simulink model "GeoSurvII_NonLinear_Signal"  (Simulink 7.3)
settings: Solver=ode23  StartTime=0.0  StopTime=30  RelTol=1e-3
values from neighbouring files (symbols this model uses):
  Uo = trim_values(10:13)    [Geo_Find_Trim.m]
  Xo = trim_values(1:9)    [Geo_Find_Trim.m]
undefined symbols (not defined in the file or in its folder): aerosimlib, Earth, sigbuilder_block, WGS
libraries: simulink x3, RCTblocks x1
settings Model: Creator=gblouin  LastModifiedBy=aholtzma
settings OptimizationCC: InitFltsAndDblsToZero=on
settings DebuggingCC: SaveWithParameterizedLinksMsg=none  SignalResolutionControl=TryResolveAllWithWarning  MultiTaskDSMMsg=warning  MultiTaskCondExecSysMsg=none
settings RTWCC: IncludeERTFirstTime=on
settings GRTTargetCC: TargetFcnLib=ansi_tfl_tmw.mat

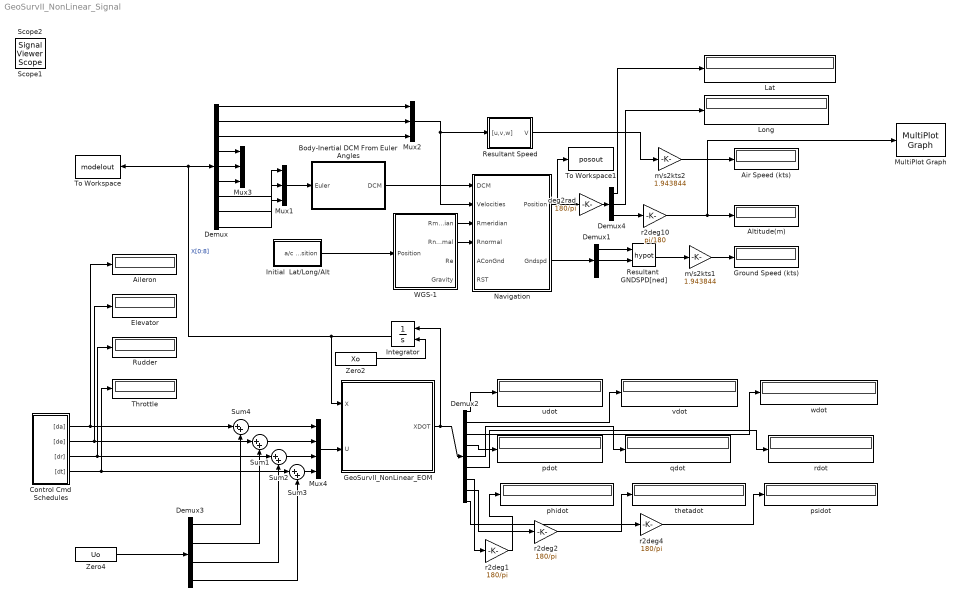
== system GeoSurvII_NonLinear_Signal ==
  Aileron : Display
  Air Speed (kts) : Display
  Altitude(m) : Display
  Body-Inertial DCM From Euler Angles : Subsystem  AncestorBlock=aerosimlib/Transformations/Body-Inertial DCM From Euler Angles
  Control Cmd Schedules : Subsystem
  Demux : Demux  Outputs=9
  Demux1 : Demux  Outputs=3
  Demux2 : Demux  Outputs=9
  Demux3 : Demux
  Demux4 : Demux  Outputs=3
  Elevator : Display
  GeoSurvII_NonLinear_EOM : Stateflow chart
  Ground Speed (kts) : Display
  Initial  Lat/Long/Alt : Subsystem
  Integrator : Integrator  InitialConditionSource=external  InitialCondition=Xo
  Lat : Display
  Long : Display
  MultiPlot Graph : RCTblocks/MultiPlot Graph  Tag=MultiPlot  SystemSampleTime=-1  tmin=0  tmax=60  ymin=450  ymax=550  Tsamp=-1  vnamesave=multisimout
  Mux1 : Mux  Inputs=3
  Mux2 : Mux  Inputs=3
  Mux3 : Mux  Inputs=3
  Mux4 : Mux
  Navigation : Subsystem
  Resultant  GNDSPD[ned] : Math  Operator=hypot  OutDataType=sfix(16)  OutScaling=2^0  SaturateOnIntegerOverflow=on
  Resultant Speed : Subsystem  AncestorBlock=aerosimlib/Equations of Motion/Body-Frame EOM/Kinematics (Euler)
  Rudder : Display
  Sum{1..4} (4 alike) : Sum  Inputs=|++  OutDataType=sfix(16)  OutScaling=2^0
  Throttle : Display
  To Workspace : ToWorkspace  VariableName=modelout  SampleTime=-1  SaveFormat=Structure
  To Workspace1 : ToWorkspace  VariableName=posout  SampleTime=-1  SaveFormat=Structure
  WGS-1 : Subsystem  AncestorBlock=aerosimlib/Earth/WGS-84
  Zero2 : Constant  Value=Xo  OutDataType=sfix(16)  OutScaling=2^0
  Zero4 : Constant  Value=Uo  OutDataType=sfix(16)  OutScaling=2^0
  deg2rad : Gain  Gain=180/pi  ParameterDataType=sfix(16)  ParameterScaling=2^0  OutDataType=sfix(16)  OutScaling=2^0
  m/s2kts1 : Gain  Gain=1.943844  ParameterDataType=sfix(16)  ParameterScaling=2^0  OutDataType=sfix(16)  OutScaling=2^0
  m/s2kts2 : Gain  Gain=1.943844  ParameterDataType=sfix(16)  ParameterScaling=2^0  OutDataType=sfix(16)  OutScaling=2^0
  pdot : Display
  phidot : Display
  psidot : Display
  qdot : Display
  r2deg1 : Gain  Gain=180/pi  ParameterDataType=sfix(16)  ParameterScaling=2^0  OutDataType=sfix(16)  OutScaling=2^0
  r2deg10 : Gain  Gain=pi/180  ParameterDataType=sfix(16)  ParameterScaling=2^0  OutDataType=sfix(16)  OutScaling=2^0
  r2deg2 : Gain  Gain=180/pi  ParameterDataType=sfix(16)  ParameterScaling=2^0  OutDataType=sfix(16)  OutScaling=2^0
  r2deg4 : Gain  Gain=180/pi  ParameterDataType=sfix(16)  ParameterScaling=2^0  OutDataType=sfix(16)  OutScaling=2^0
  rdot : Display
  thetadot : Display
  udot : Display
  vdot : Display
  wdot : Display
  Scope1 : SignalViewerScope  IOType=viewer  NumInputPorts=2  ZoomMode=xonly  RefreshTime=1.500000
      settings: TimeRange=100  YMin=-3.5~-2.84987e-012  YMax=0.5~-2.57845e-012  MaxDataPoints=20000
  Scope2 : SignalViewerScope  IOType=viewer  NumInputPorts=2  ZoomMode=xonly  RefreshTime=1.500000
      settings: TimeRange=100  YMin=-40~9.16954  YMax=10~10.1348  MaxDataPoints=20000
  wires:
  Navigation/1(Position) -> deg2rad/1, To Workspace1/1
  Demux4/1 -> Lat/1
  Demux4/2 -> Long/1
  deg2rad/1 -> Demux4/1
  Demux4/3 -> r2deg10/1
  r2deg10/1 -> Altitude(m)/1, MultiPlot Graph/1
  Navigation/2(Gndspd) -> Demux1/1
  Demux1/1 -> Resultant  GNDSPD[ned]/1
  Demux1/2 -> Resultant  GNDSPD[ned]/2
  Integrator/1 -> GeoSurvII_NonLinear_EOM/1(X), Demux/1, To Workspace/1  "X[0:8]"
  Zero2/1 -> Integrator/2
  Demux2/2 -> vdot/1
  Demux2/1 -> udot/1
  GeoSurvII_NonLinear_EOM/1(XDOT) -> Demux2/1, Integrator/1
  Zero4/1 -> Demux3/1
  Mux4/1 -> GeoSurvII_NonLinear_EOM/2(U)
  Demux/1 -> Mux2/1
  Resultant  GNDSPD[ned]/1 -> m/s2kts1/1
  m/s2kts1/1 -> Ground Speed (kts)/1
  WGS-1/1(Rmeridian) -> Navigation/3(Rmeridian)
  WGS-1/2(Rnormal) -> Navigation/4(Rnormal)
  Body-Inertial DCM From Euler Angles/1(DCM) -> Navigation/1(DCM)
  Mux2/1 -> Navigation/2(Velocities), Resultant Speed/1("[u,v,w]")
  Initial  Lat/Long/Alt/1(a/c Position) -> WGS-1/1(Position)
  Resultant Speed/1(V) -> m/s2kts2/1
  m/s2kts2/1 -> Air Speed (kts)/1
  Demux2/3 -> wdot/1
  Demux2/4 -> pdot/1
  Demux2/5 -> qdot/1
  Demux2/6 -> rdot/1
  Demux2/7 -> r2deg1/1
  r2deg1/1 -> phidot/1
  Demux2/8 -> r2deg2/1
  r2deg2/1 -> thetadot/1
  Demux2/9 -> r2deg4/1
  r2deg4/1 -> psidot/1
  Sum4/1 -> Mux4/1
  Sum1/1 -> Mux4/2
  Sum2/1 -> Mux4/3
  Sum3/1 -> Mux4/4
  Demux3/1 -> Sum4/2
  Demux3/2 -> Sum1/2
  Demux3/3 -> Sum2/2
  Demux3/4 -> Sum3/2
  Demux/2 -> Mux2/2
  Demux/3 -> Mux2/3
  Demux/7 -> Mux1/1
  Demux/8 -> Mux1/2
  Demux/9 -> Mux1/3
  Mux1/1 -> Body-Inertial DCM From Euler Angles/1(Euler)
  Demux/4 -> Mux3/1
  Demux/5 -> Mux3/2
  Demux/6 -> Mux3/3
  Control Cmd Schedules/1("[da]") -> Sum4/1, Aileron/1
  Control Cmd Schedules/2("[de]") -> Sum1/1, Elevator/1
  Control Cmd Schedules/3("[dr]") -> Sum2/1, Rudder/1
  Control Cmd Schedules/4("[dt]") -> Sum3/1, Throttle/1

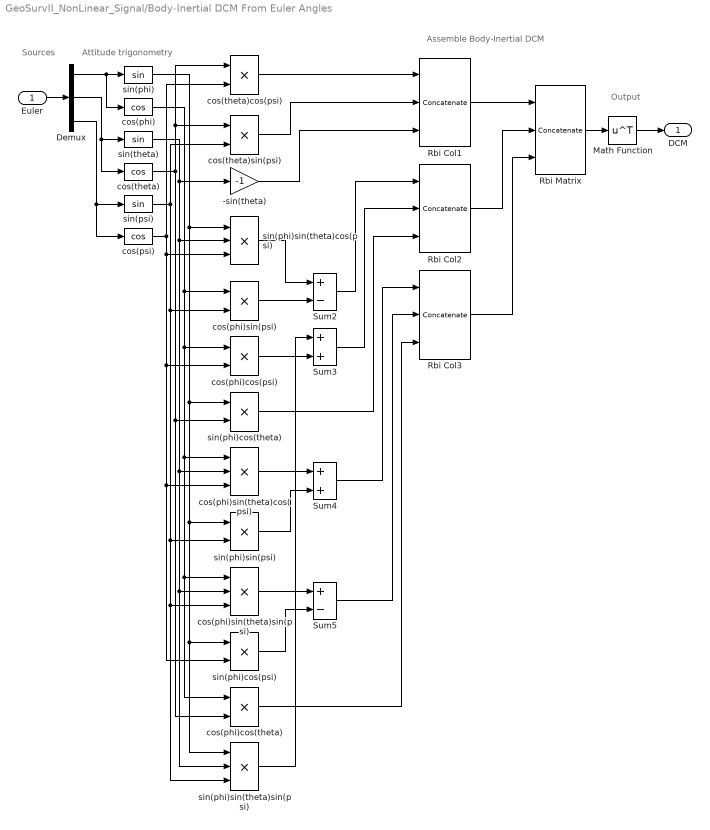
== system GeoSurvII_NonLinear_Signal/Body-Inertial DCM From Euler Angles ==
  note: Sources
  note: Assemble Body-Inertial DCM
  note: Output
  note: Attitude trigonometry
  Euler : Inport  PortDimensions=[3 1]  OutDataType=sfix(16)  OutScaling=2^0
  -sin(theta) : Gain  Gain=-1  ParameterDataType=sfix(16)  ParameterScaling=2^0  OutDataType=sfix(16)  OutScaling=2^0  SaturateOnIntegerOverflow=on  OutDataTypeStr=Inherit: Same as input  ParamDataTypeStr=Inherit: Same as input
  Demux : Demux  Outputs=3
  Math Function : Math  Operator=transpose  OutDataType=sfix(16)  OutScaling=2^0  SaturateOnIntegerOverflow=on
  Rbi Matrix : Concatenate  NumInputs=3  Mode=Multidimensional array  ConcatenateDimension=2
  Rbi Col1 : Concatenate  NumInputs=3  Mode=Multidimensional array
  Rbi Col2 : Concatenate  NumInputs=3  Mode=Multidimensional array
  Rbi Col3 : Concatenate  NumInputs=3  Mode=Multidimensional array
  Sum2 : Sum  Inputs=+-  OutDataType=sfix(16)  OutScaling=2^0  SaturateOnIntegerOverflow=on  InputSameDT=on  OutDataTypeStr=Inherit: Same as first input
  Sum3 : Sum  OutDataType=sfix(16)  OutScaling=2^0  SaturateOnIntegerOverflow=on  InputSameDT=on  OutDataTypeStr=Inherit: Same as first input
  Sum4 : Sum  OutDataType=sfix(16)  OutScaling=2^0  SaturateOnIntegerOverflow=on  InputSameDT=on  OutDataTypeStr=Inherit: Same as first input
  Sum5 : Sum  Inputs=+-  OutDataType=sfix(16)  OutScaling=2^0  SaturateOnIntegerOverflow=on  InputSameDT=on  OutDataTypeStr=Inherit: Same as first input
  cos(phi) : Trigonometry  Operator=cos
  cos(phi)cos(psi) : Product  OutDataType=sfix(16)  OutScaling=2^0  SaturateOnIntegerOverflow=on  InputSameDT=on  OutDataTypeStr=Inherit: Same as first input
  cos(phi)cos(theta) : Product  OutDataType=sfix(16)  OutScaling=2^0  SaturateOnIntegerOverflow=on  InputSameDT=on  OutDataTypeStr=Inherit: Same as first input
  cos(phi)sin(psi) : Product  OutDataType=sfix(16)  OutScaling=2^0  SaturateOnIntegerOverflow=on  InputSameDT=on  OutDataTypeStr=Inherit: Same as first input
  cos(phi)sin(theta)cos(psi) : Product  Inputs=3  OutDataType=sfix(16)  OutScaling=2^0  SaturateOnIntegerOverflow=on  InputSameDT=on  OutDataTypeStr=Inherit: Same as first input
  cos(phi)sin(theta)sin(psi) : Product  Inputs=3  OutDataType=sfix(16)  OutScaling=2^0  SaturateOnIntegerOverflow=on  InputSameDT=on  OutDataTypeStr=Inherit: Same as first input
  cos(psi) : Trigonometry  Operator=cos
  cos(theta) : Trigonometry  Operator=cos
  cos(theta)cos(psi) : Product  OutDataType=sfix(16)  OutScaling=2^0  SaturateOnIntegerOverflow=on  InputSameDT=on  OutDataTypeStr=Inherit: Same as first input
  cos(theta)sin(psi) : Product  OutDataType=sfix(16)  OutScaling=2^0  SaturateOnIntegerOverflow=on  InputSameDT=on  OutDataTypeStr=Inherit: Same as first input
  sin(phi) : Trigonometry
  sin(phi)cos(psi) : Product  OutDataType=sfix(16)  OutScaling=2^0  SaturateOnIntegerOverflow=on  InputSameDT=on  OutDataTypeStr=Inherit: Same as first input
  sin(phi)cos(theta) : Product  OutDataType=sfix(16)  OutScaling=2^0  SaturateOnIntegerOverflow=on  InputSameDT=on  OutDataTypeStr=Inherit: Same as first input
  sin(phi)sin(psi) : Product  OutDataType=sfix(16)  OutScaling=2^0  SaturateOnIntegerOverflow=on  InputSameDT=on  OutDataTypeStr=Inherit: Same as first input
  sin(phi)sin(theta)cos(psi) : Product  Inputs=3  OutDataType=sfix(16)  OutScaling=2^0  SaturateOnIntegerOverflow=on  InputSameDT=on  OutDataTypeStr=Inherit: Same as first input
  sin(phi)sin(theta)sin(psi) : Product  Inputs=3  OutDataType=sfix(16)  OutScaling=2^0  SaturateOnIntegerOverflow=on  InputSameDT=on  OutDataTypeStr=Inherit: Same as first input
  sin(psi) : Trigonometry
  sin(theta) : Trigonometry
  DCM : Outport  OutDataType=sfix(16)  OutScaling=2^0
  wires:
  Euler/1 -> Demux/1
  Rbi Col1/1 -> Rbi Matrix/1
  Rbi Col2/1 -> Rbi Matrix/2
  Rbi Col3/1 -> Rbi Matrix/3
  Rbi Matrix/1 -> Math Function/1
  Demux/1 -> sin(phi)/1, cos(phi)/1
  Demux/2 -> cos(theta)/1, sin(theta)/1
  Demux/3 -> cos(psi)/1, sin(psi)/1
  sin(phi)/1 -> sin(phi)sin(psi)/1, sin(phi)cos(psi)/1, sin(phi)sin(theta)sin(psi)/1, sin(phi)cos(theta)/1, sin(phi)sin(theta)cos(psi)/1
  cos(phi)/1 -> cos(phi)cos(theta)/1, cos(phi)sin(theta)sin(psi)/1, cos(phi)sin(theta)cos(psi)/1, cos(phi)cos(psi)/1, cos(phi)sin(psi)/1
  sin(theta)/1 -> cos(phi)sin(theta)cos(psi)/2, cos(phi)sin(theta)sin(psi)/2, sin(phi)sin(theta)sin(psi)/2, sin(phi)sin(theta)cos(psi)/2, -sin(theta)/1
  cos(theta)/1 -> cos(phi)cos(theta)/2, sin(phi)cos(theta)/2, cos(theta)sin(psi)/1, cos(theta)cos(psi)/1
  sin(psi)/1 -> sin(phi)sin(psi)/2, cos(phi)sin(theta)sin(psi)/3, sin(phi)sin(theta)sin(psi)/3, cos(phi)sin(psi)/2, cos(theta)sin(psi)/2
  cos(psi)/1 -> sin(phi)cos(psi)/2, cos(phi)sin(theta)cos(psi)/3, cos(phi)cos(psi)/2, sin(phi)sin(theta)cos(psi)/3, cos(theta)cos(psi)/2
  cos(phi)sin(psi)/1 -> Sum2/2
  cos(phi)cos(psi)/1 -> Sum3/2
  sin(phi)sin(theta)cos(psi)/1 -> Sum2/1
  cos(phi)sin(theta)cos(psi)/1 -> Sum4/1
  sin(phi)sin(psi)/1 -> Sum4/2
  cos(phi)sin(theta)sin(psi)/1 -> Sum5/1
  sin(phi)cos(psi)/1 -> Sum5/2
  cos(theta)cos(psi)/1 -> Rbi Col1/1
  cos(theta)sin(psi)/1 -> Rbi Col1/2
  -sin(theta)/1 -> Rbi Col1/3
  Sum2/1 -> Rbi Col2/1
  Sum3/1 -> Rbi Col2/2
  sin(phi)cos(theta)/1 -> Rbi Col2/3
  Sum4/1 -> Rbi Col3/1
  Sum5/1 -> Rbi Col3/2
  cos(phi)cos(theta)/1 -> Rbi Col3/3
  Math Function/1 -> DCM/1
  sin(phi)sin(theta)sin(psi)/1 -> Sum3/1

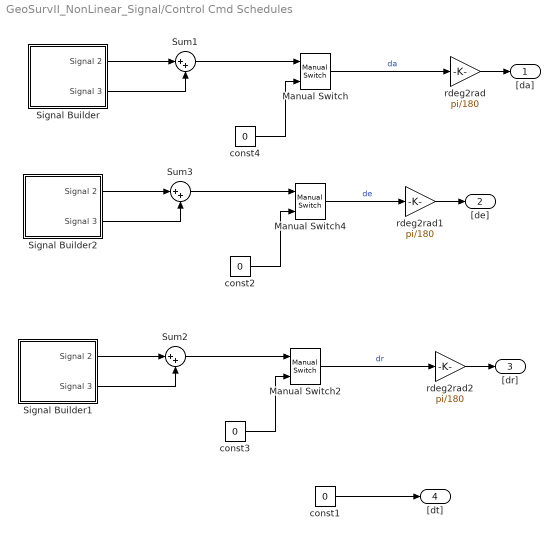
== system GeoSurvII_NonLinear_Signal/Control Cmd Schedules ==
  Manual Switch : simulink/Signal Routing/Manual Switch  SystemSampleTime=-1  sw=0  action=0  varsize=off
  Manual Switch2 : simulink/Signal Routing/Manual Switch  SystemSampleTime=-1  sw=0  action=0  varsize=off
  Manual Switch4 : simulink/Signal Routing/Manual Switch  SystemSampleTime=-1  sw=0  action=0  varsize=off
  Signal Builder : Subsystem  Tag=STV Subsys  LoadFcn=sigbuilder_block('load');  StartFcn=sigbuilder_block('start');  StopFcn=sigbuilder_block('stop');  ClipboardFcn=sigbuilder_block('clipboard');  mask(Sigbuilder block){}
      mask help: Sigbuilder GUI
      mask init:
      | if ~strcmp(get_param(bdroot(gcbh),'SimulationStatus'),'stopped') tuvar = sigbuilder_block('maskInit'); end
      settings: CopyFcn=sigbuilder_block('copy');  DeleteFcn=sigbuilder_block('delete');  ModelCloseFcn=sigbuilder_block('modelClose');  PreSaveFcn=sigbuilder_block('preSave');  NameChangeFcn=sigbuilder_block('namechange');  OpenFcn=sigbuilder_block('open',[6 22.5 948 659.25 ]);  CloseFcn=sigbuilder_block('close');
      mask Display: plot(0,0,100,100,[10,10,40,40,10],[80,20,20,80,80],[40,10],[50,50], [40,27,10],[65,72,56],[40,25,25,10],[28,28,43,43]);
  Signal Builder1 : Subsystem  Tag=STV Subsys  LoadFcn=sigbuilder_block('load');  StartFcn=sigbuilder_block('start');  StopFcn=sigbuilder_block('stop');  ClipboardFcn=sigbuilder_block('clipboard');  mask(Sigbuilder block){}
      mask help: Sigbuilder GUI
      mask init:
      | if ~strcmp(get_param(bdroot(gcbh),'SimulationStatus'),'stopped') tuvar = sigbuilder_block('maskInit'); end
      settings: CopyFcn=sigbuilder_block('copy');  DeleteFcn=sigbuilder_block('delete');  ModelCloseFcn=sigbuilder_block('modelClose');  PreSaveFcn=sigbuilder_block('preSave');  NameChangeFcn=sigbuilder_block('namechange');  OpenFcn=sigbuilder_block('open',[0 19.5 960 695.25 ]);  CloseFcn=sigbuilder_block('close');
      mask Display: plot(0,0,100,100,[10,10,40,40,10],[80,20,20,80,80],[40,10],[50,50], [40,27,10],[65,72,56],[40,25,25,10],[28,28,43,43]);
  Signal Builder2 : Subsystem  Tag=STV Subsys  LoadFcn=sigbuilder_block('load');  StartFcn=sigbuilder_block('start');  StopFcn=sigbuilder_block('stop');  ClipboardFcn=sigbuilder_block('clipboard');  mask(Sigbuilder block){}
      mask help: Sigbuilder GUI
      mask init:
      | if ~strcmp(get_param(bdroot(gcbh),'SimulationStatus'),'stopped') tuvar = sigbuilder_block('maskInit'); end
      settings: CopyFcn=sigbuilder_block('copy');  DeleteFcn=sigbuilder_block('delete');  ModelCloseFcn=sigbuilder_block('modelClose');  PreSaveFcn=sigbuilder_block('preSave');  NameChangeFcn=sigbuilder_block('namechange');  OpenFcn=sigbuilder_block('open',[6 22.5 948 659.25 ]);  CloseFcn=sigbuilder_block('close');
      mask Display: plot(0,0,100,100,[10,10,40,40,10],[80,20,20,80,80],[40,10],[50,50], [40,27,10],[65,72,56],[40,25,25,10],[28,28,43,43]);
  Sum1 : Sum  Inputs=|++  OutDataType=sfix(16)  OutScaling=2^0
  Sum2 : Sum  Inputs=|++  OutDataType=sfix(16)  OutScaling=2^0
  Sum3 : Sum  Inputs=|++  OutDataType=sfix(16)  OutScaling=2^0
  const{1..4} (4 alike) : Constant  Value=0  OutDataType=sfix(16)  OutScaling=2^0
  rdeg2rad : Gain  Gain=pi/180  ParameterDataType=sfix(16)  ParameterScaling=2^0  OutDataType=sfix(16)  OutScaling=2^0
  rdeg2rad1 : Gain  Gain=pi/180  ParameterDataType=sfix(16)  ParameterScaling=2^0  OutDataType=sfix(16)  OutScaling=2^0
  rdeg2rad2 : Gain  Gain=pi/180  ParameterDataType=sfix(16)  ParameterScaling=2^0  OutDataType=sfix(16)  OutScaling=2^0
  "[da]" : Outport  OutDataType=sfix(16)  OutScaling=2^0
  "[de]" : Outport  Port=2  OutDataType=sfix(16)  OutScaling=2^0
  "[dr]" : Outport  Port=3  OutDataType=sfix(16)  OutScaling=2^0
  "[dt]" : Outport  Port=4  OutDataType=sfix(16)  OutScaling=2^0
  wires:
  Signal Builder/1(Signal 2) -> Sum1/1
  Signal Builder/2(Signal 3) -> Sum1/2
  Manual Switch/1 -> rdeg2rad/1  "da"
  Sum1/1 -> Manual Switch/1
  const4/1 -> Manual Switch/2
  Signal Builder1/1(Signal 2) -> Sum2/1
  Signal Builder1/2(Signal 3) -> Sum2/2
  Manual Switch2/1 -> rdeg2rad2/1  "dr"
  Sum2/1 -> Manual Switch2/1
  const3/1 -> Manual Switch2/2
  Signal Builder2/1(Signal 2) -> Sum3/1
  Signal Builder2/2(Signal 3) -> Sum3/2
  Manual Switch4/1 -> rdeg2rad1/1  "de"
  Sum3/1 -> Manual Switch4/1
  const2/1 -> Manual Switch4/2
  const1/1 -> "[dt]"/1
  rdeg2rad/1 -> "[da]"/1
  rdeg2rad1/1 -> "[de]"/1
  rdeg2rad2/1 -> "[dr]"/1

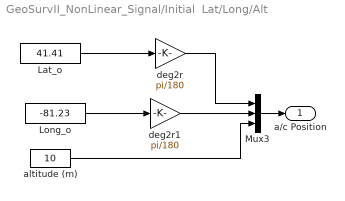
== system GeoSurvII_NonLinear_Signal/Initial  Lat/Long/Alt ==
  Lat_o : Constant  Value=41.41  OutDataType=sfix(16)  OutScaling=2^0
  Long_o : Constant  Value=-81.23  OutDataType=sfix(16)  OutScaling=2^0
  Mux3 : Mux  Inputs=3
  altitude (m) : Constant  Value=10  OutDataType=sfix(16)  OutScaling=2^0
  deg2r : Gain  Gain=pi/180  ParameterDataType=sfix(16)  ParameterScaling=2^0  OutDataType=sfix(16)  OutScaling=2^0
  deg2r1 : Gain  Gain=pi/180  ParameterDataType=sfix(16)  ParameterScaling=2^0  OutDataType=sfix(16)  OutScaling=2^0
  a/c Position : Outport  OutDataType=sfix(16)  OutScaling=2^0
  wires:
  Mux3/1 -> a/c Position/1
  altitude (m)/1 -> Mux3/3
  deg2r1/1 -> Mux3/2
  deg2r/1 -> Mux3/1
  Long_o/1 -> deg2r1/1
  Lat_o/1 -> deg2r/1

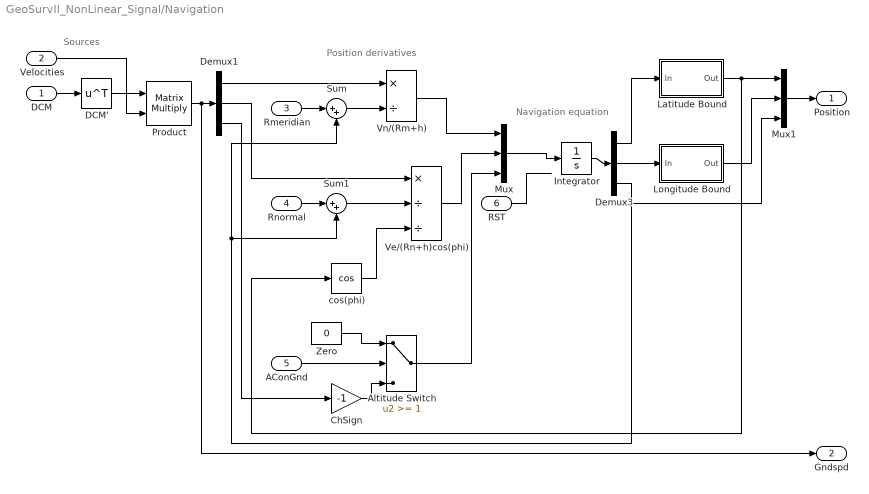
== system GeoSurvII_NonLinear_Signal/Navigation ==
  note: Navigation equation
  note: Position derivatives
  note: Sources
  DCM : Inport  PortDimensions=[3 3]  OutDataType=sfix(16)  OutScaling=2^0
  Velocities : Inport  Port=2  PortDimensions=[3 1]  OutDataType=sfix(16)  OutScaling=2^0
  Rmeridian : Inport  Port=3  PortDimensions=1  OutDataType=sfix(16)  OutScaling=2^0
  Rnormal : Inport  Port=4  PortDimensions=1  OutDataType=sfix(16)  OutScaling=2^0
  AConGnd : Inport  Port=5  PortDimensions=1  OutDataType=sfix(16)  OutScaling=2^0
  RST : Inport  Port=6  PortDimensions=1  OutDataType=sfix(16)  OutScaling=2^0
  Altitude Switch : Switch  Threshold=1  SaturateOnIntegerOverflow=on  InputSameDT=on
  ChSign : Gain  Gain=-1  ParameterDataType=sfix(16)  ParameterScaling=2^0  OutDataType=sfix(16)  OutScaling=2^0  SaturateOnIntegerOverflow=on  OutDataTypeStr=Inherit: Same as input  ParamDataTypeStr=Inherit: Same as input
  DCM' : Math  Operator=transpose  OutDataType=sfix(16)  OutScaling=2^0  SaturateOnIntegerOverflow=on
  Demux1 : Demux  Outputs=3
  Demux3 : Demux  Outputs=3
  Integrator : Integrator  InitialCondition=[41.684028*pi/180 -81.389750*pi/180 500]
  Latitude Bound : Subsystem
      mask Type: Latitude bound
      mask Description: Bounds the latitude to [-pi/2, pi/2]. When the lower bound is exceeded the latitude is increasing again; when the upper bound is exceeded the latitude is decreasing.
  Longitude Bound : Subsystem
      mask Type: Longitude bound
      mask Description: Bounds the longitude to [-pi, pi]. When -pi bound is exceeded the longitude wraps back to pi; when the pi bound is exceeded the longitude wraps back to -pi.
  Mux : Mux  Inputs=3
  Mux1 : Mux  Inputs=3
  Product : Product  Multiplication=Matrix(*)  OutDataType=sfix(16)  OutScaling=2^0  SaturateOnIntegerOverflow=on  InputSameDT=on  OutDataTypeStr=Inherit: Same as first input
  Sum : Sum  Inputs=|++  OutDataType=sfix(16)  OutScaling=2^0  SaturateOnIntegerOverflow=on  InputSameDT=on  OutDataTypeStr=Inherit: Same as first input
  Sum1 : Sum  Inputs=|++  OutDataType=sfix(16)  OutScaling=2^0  SaturateOnIntegerOverflow=on  InputSameDT=on  OutDataTypeStr=Inherit: Same as first input
  Ve/(Rn+h)cos(phi) : Product  Inputs=*//  OutDataType=sfix(16)  OutScaling=2^0  SaturateOnIntegerOverflow=on  InputSameDT=on  OutDataTypeStr=Inherit: Same as first input
  Vn/(Rm+h) : Product  Inputs=*/  OutDataType=sfix(16)  OutScaling=2^0  SaturateOnIntegerOverflow=on  InputSameDT=on  OutDataTypeStr=Inherit: Same as first input
  Zero : Constant  Value=0  OutDataType=sfix(16)  OutScaling=2^0
  cos(phi) : Trigonometry  Operator=cos
  Position : Outport  OutDataType=sfix(16)  OutScaling=2^0
  Gndspd : Outport  Port=2  OutDataType=sfix(16)  OutScaling=2^0
  wires:
  Latitude Bound/1(Out) -> Mux1/1, cos(phi)/1
  Mux1/1 -> Position/1
  Longitude Bound/1(Out) -> Mux1/2
  Demux3/1 -> Latitude Bound/1(In)
  Demux3/2 -> Longitude Bound/1(In)
  Demux3/3 -> Mux1/3, Sum1/2, Sum/2
  cos(phi)/1 -> Ve/(Rn+h)cos(phi)/3
  Integrator/1 -> Demux3/1
  RST/1 -> ?
  Mux/1 -> Integrator/1
  Altitude Switch/1 -> Mux/3
  ChSign/1 -> Altitude Switch/3
  Zero/1 -> Altitude Switch/1
  AConGnd/1 -> Altitude Switch/2
  DCM'/1 -> Product/1
  DCM/1 -> DCM'/1
  Ve/(Rn+h)cos(phi)/1 -> Mux/2
  Sum1/1 -> Ve/(Rn+h)cos(phi)/2
  Vn/(Rm+h)/1 -> Mux/1
  Sum/1 -> Vn/(Rm+h)/2
  Rnormal/1 -> Sum1/1
  Rmeridian/1 -> Sum/1
  Product/1 -> Gndspd/1, Demux1/1
  Demux1/2 -> Ve/(Rn+h)cos(phi)/1
  Demux1/3 -> ChSign/1
  Demux1/1 -> Vn/(Rm+h)/1
  Velocities/1 -> Product/2

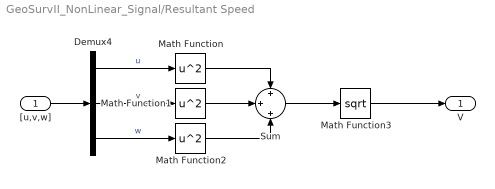
== system GeoSurvII_NonLinear_Signal/Resultant Speed ==
  "[u,v,w]" : Inport  PortDimensions=[3 1]  OutDataType=sfix(16)  OutScaling=2^0
  Demux4 : Demux  Outputs=3
  Math Function : Math  Operator=square  OutDataType=sfix(16)  OutScaling=2^0  SaturateOnIntegerOverflow=on
  Math Function1 : Math  Operator=square  OutDataType=sfix(16)  OutScaling=2^0  SaturateOnIntegerOverflow=on
  Math Function2 : Math  Operator=square  OutDataType=sfix(16)  OutScaling=2^0  SaturateOnIntegerOverflow=on
  Math Function3 : Math  Operator=sqrt  OutDataType=sfix(16)  OutScaling=2^0  SaturateOnIntegerOverflow=on
  Sum : Sum  Inputs=+|+|+  OutDataType=sfix(16)  OutScaling=2^0
  V : Outport  OutDataType=sfix(16)  OutScaling=2^0
  wires:
  Demux4/2 -> Math Function1/1  "v"
  Demux4/3 -> Math Function2/1  "w"
  Math Function/1 -> Sum/1
  Math Function1/1 -> Sum/2
  Math Function2/1 -> Sum/3
  Sum/1 -> Math Function3/1
  Math Function3/1 -> V/1
  Demux4/1 -> Math Function/1  "u"
  "[u,v,w]"/1 -> Demux4/1

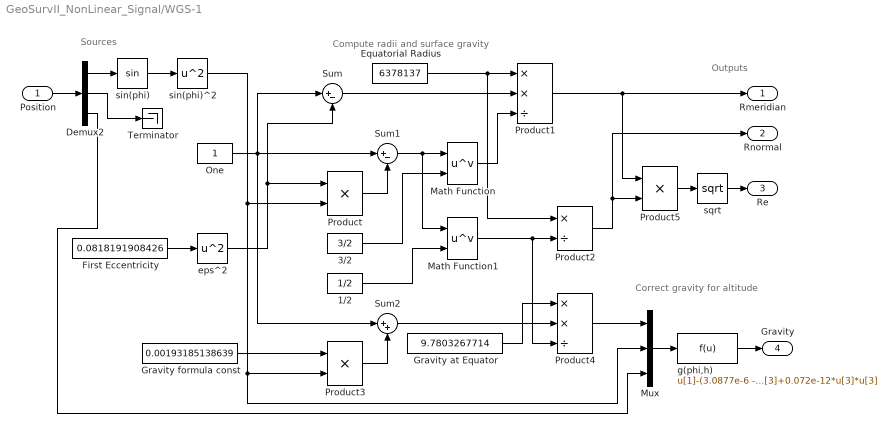
== system GeoSurvII_NonLinear_Signal/WGS-1 ==
  note: Sources
  note: Compute radii and surface gravity
  note: Correct gravity for altitude
  note: Outputs
  Position : Inport  OutDataType=sfix(16)  OutScaling=2^0
  1/2 : Constant  Value=1/2  OutDataType=sfix(16)  OutScaling=2^0
  3/2 : Constant  Value=3/2  OutDataType=sfix(16)  OutScaling=2^0
  Demux2 : Demux  Outputs=3
  Equatorial Radius : Constant  Value=6378137  OutDataType=sfix(16)  OutScaling=2^0
  First Eccentricity : Constant  Value=0.0818191908426  OutDataType=sfix(16)  OutScaling=2^0
  Gravity at Equator : Constant  Value=9.7803267714  OutDataType=sfix(16)  OutScaling=2^0
  Gravity formula const : Constant  Value=0.00193185138639  OutDataType=sfix(16)  OutScaling=2^0
  Math Function : Math  Operator=pow  OutDataType=sfix(16)  OutScaling=2^0  SaturateOnIntegerOverflow=on
  Math Function1 : Math  Operator=pow  OutDataType=sfix(16)  OutScaling=2^0  SaturateOnIntegerOverflow=on
  Mux : Mux  Inputs=3
  One : Constant  OutDataType=sfix(16)  OutScaling=2^0
  Product : Product  OutDataType=sfix(16)  OutScaling=2^0  SaturateOnIntegerOverflow=on  InputSameDT=on  OutDataTypeStr=Inherit: Same as first input
  Product1 : Product  Inputs=**/  OutDataType=sfix(16)  OutScaling=2^0  SaturateOnIntegerOverflow=on  InputSameDT=on  OutDataTypeStr=Inherit: Same as first input
  Product2 : Product  Inputs=*/  OutDataType=sfix(16)  OutScaling=2^0  SaturateOnIntegerOverflow=on  InputSameDT=on  OutDataTypeStr=Inherit: Same as first input
  Product3 : Product  OutDataType=sfix(16)  OutScaling=2^0  SaturateOnIntegerOverflow=on  InputSameDT=on  OutDataTypeStr=Inherit: Same as first input
  Product4 : Product  Inputs=**/  OutDataType=sfix(16)  OutScaling=2^0  SaturateOnIntegerOverflow=on  InputSameDT=on  OutDataTypeStr=Inherit: Same as first input
  Product5 : Product  OutDataType=sfix(16)  OutScaling=2^0  SaturateOnIntegerOverflow=on  InputSameDT=on  OutDataTypeStr=Inherit: Same as first input
  Sum : Sum  Inputs=|+-  OutDataType=sfix(16)  OutScaling=2^0  SaturateOnIntegerOverflow=on  InputSameDT=on  OutDataTypeStr=Inherit: Same as first input
  Sum1 : Sum  Inputs=|+-  OutDataType=sfix(16)  OutScaling=2^0  SaturateOnIntegerOverflow=on  InputSameDT=on  OutDataTypeStr=Inherit: Same as first input
  Sum2 : Sum  Inputs=|++  OutDataType=sfix(16)  OutScaling=2^0  SaturateOnIntegerOverflow=on  InputSameDT=on  OutDataTypeStr=Inherit: Same as first input
  Terminator : Terminator
  eps^2 : Math  Operator=square  OutDataType=sfix(16)  OutScaling=2^0  SaturateOnIntegerOverflow=on
  g(phi,h) : Fcn  Expr=u[1]-(3.0877e-6 - 0.0044e-6*u[2])*u[3]+0.072e-12*u[3]*u[3]
  sin(phi) : Trigonometry
  sin(phi)^2 : Math  Operator=square  OutDataType=sfix(16)  OutScaling=2^0  SaturateOnIntegerOverflow=on
  sqrt : Math  Operator=sqrt  OutDataType=sfix(16)  OutScaling=2^0  SaturateOnIntegerOverflow=on
  Rmeridian : Outport  OutDataType=sfix(16)  OutScaling=2^0
  Rnormal : Outport  Port=2  OutDataType=sfix(16)  OutScaling=2^0
  Re : Outport  Port=3  OutDataType=sfix(16)  OutScaling=2^0
  Gravity : Outport  Port=4  OutDataType=sfix(16)  OutScaling=2^0
  wires:
  sqrt/1 -> Re/1
  Product5/1 -> sqrt/1
  First Eccentricity/1 -> eps^2/1
  eps^2/1 -> Sum/2, Product/1
  sin(phi)/1 -> sin(phi)^2/1
  sin(phi)^2/1 -> Product/2, Product3/2, Mux/2
  One/1 -> Sum1/1, Sum2/1, Sum/1
  Product/1 -> Sum1/2
  Sum1/1 -> Math Function/1, Math Function1/1
  3/2/1 -> Math Function/2
  1/2/1 -> Math Function1/2
  Equatorial Radius/1 -> Product1/1, Product2/1
  Sum/1 -> Product1/2
  Math Function/1 -> Product1/3
  Math Function1/1 -> Product2/2, Product4/3
  Product1/1 -> Rmeridian/1, Product5/1
  Product2/1 -> Rnormal/1, Product5/2
  Gravity formula const/1 -> Product3/1
  Product3/1 -> Sum2/2
  Gravity at Equator/1 -> Product4/1
  Sum2/1 -> Product4/2
  Product4/1 -> Mux/1
  Position/1 -> Demux2/1
  Demux2/1 -> sin(phi)/1
  Demux2/2 -> Terminator/1
  Mux/1 -> g(phi,h)/1
  g(phi,h)/1 -> Gravity/1
  Demux2/3 -> Mux/3

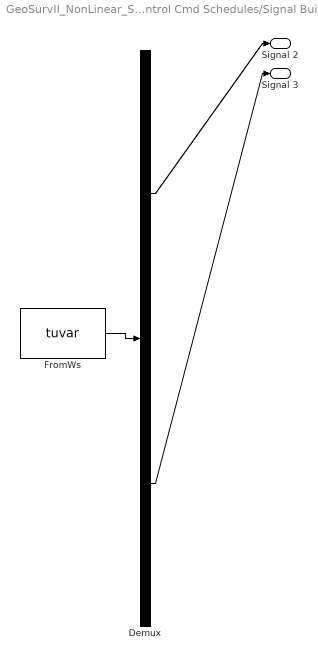
== system GeoSurvII_NonLinear_Signal/Control Cmd Schedules/Signal Builder ==
  Demux : Demux  Tag=STV Demux  Outputs=2
  FromWs : FromWorkspace  Tag=STV FromWs  VariableName=tuvar  SampleTime=0  SigBuilderData=DataTag0  VnvData=DataTag1
      SigBuilderData=|
      | channels(1).label = 'Signal 2'
      | channels(1).allXData = {[0 1 1 15 60]}
      | channels(1).allYData = {[5 5 0 0 0]}
      | channels(2).label = 'Signal 3'
      | channels(2).allXData = {[0 1 1 2 2 60]}
      | channels(2).allYData = {[0 0 -5 -5 0 0]}
      | common.afterFinalStr = 'Extrapolate'
      | common.sampleTime = 0
      | dataSet.timeRange = [0 60]
      | dataSet.name = 'Group 1'
  Signal 2 : Outport  Tag=STV Outport  OutDataType=sfix(16)  OutScaling=2^0
  Signal 3 : Outport  Tag=STV Outport  Port=2  OutDataType=sfix(16)  OutScaling=2^0
  wires:
  Demux/1 -> Signal 2/1
  FromWs/1 -> Demux/1
  Demux/2 -> Signal 3/1

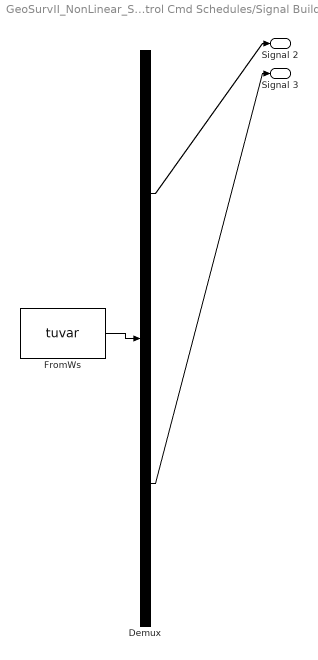
== system GeoSurvII_NonLinear_Signal/Control Cmd Schedules/Signal Builder1 ==
  Demux : Demux  Tag=STV Demux  Outputs=2
  FromWs : FromWorkspace  Tag=STV FromWs  VariableName=tuvar  SampleTime=0  SigBuilderData=DataTag2  VnvData=DataTag3
      SigBuilderData=|
      | channels(1).label = 'Signal 2'
      | channels(1).allXData = {[0 1 1 15 60]}
      | channels(1).allYData = {[1 1 0 0 0]}
      | channels(2).label = 'Signal 3'
      | channels(2).allXData = {[0 3 3.9 60]}
      | channels(2).allYData = {[0 0 0 0]}
      | common.afterFinalStr = 'Extrapolate'
      | common.sampleTime = 0
      | dataSet.timeRange = [0 60]
      | dataSet.name = 'Group 1'
  Signal 2 : Outport  Tag=STV Outport  OutDataType=sfix(16)  OutScaling=2^0
  Signal 3 : Outport  Tag=STV Outport  Port=2  OutDataType=sfix(16)  OutScaling=2^0
  wires:
  Demux/1 -> Signal 2/1
  FromWs/1 -> Demux/1
  Demux/2 -> Signal 3/1

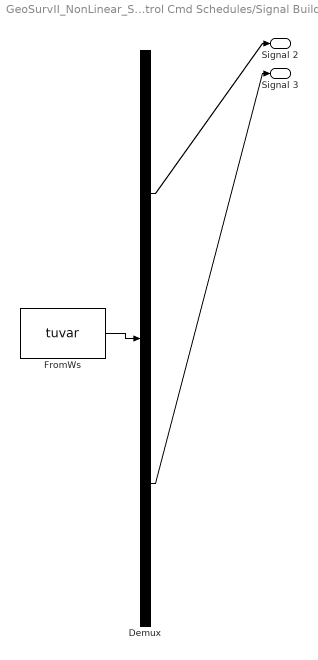
== system GeoSurvII_NonLinear_Signal/Control Cmd Schedules/Signal Builder2 ==
  Demux : Demux  Tag=STV Demux  Outputs=2
  FromWs : FromWorkspace  Tag=STV FromWs  VariableName=tuvar  SampleTime=0  SigBuilderData=DataTag4  VnvData=DataTag5
      SigBuilderData=|
      | common.afterFinalStr = 'Extrapolate'
      | common.sampleTime = 0
      | dataSet.timeRange = [0 60]
      | dataSet.name = 'Group 1'
      | sbobj.Groups{1}.Signals{1}.XData = [0 1 1 2 2 60]
      | sbobj.Groups{1}.Signals{1}.YData = [0 0 1 1 0 0]
      | sbobj.Groups{1}.Signals{2}.XData = [0 2 2 3 3 60]
      | sbobj.Groups{1}.Signals{2}.YData = [0 0 -1 -1 0 0]
  Signal 2 : Outport  Tag=STV Outport  OutDataType=sfix(16)  OutScaling=2^0
  Signal 3 : Outport  Tag=STV Outport  Port=2  OutDataType=sfix(16)  OutScaling=2^0
  wires:
  Demux/1 -> Signal 2/1
  FromWs/1 -> Demux/1
  Demux/2 -> Signal 3/1

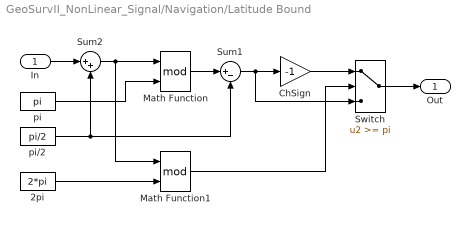
== system GeoSurvII_NonLinear_Signal/Navigation/Latitude Bound ==
  In : Inport  OutDataType=sfix(16)  OutScaling=2^0
  2pi : Constant  Value=2*pi  OutDataType=sfix(16)  OutScaling=2^0
  ChSign : Gain  Gain=-1  ParameterDataType=sfix(16)  ParameterScaling=2^0  OutDataType=sfix(16)  OutScaling=2^0  SaturateOnIntegerOverflow=on  OutDataTypeStr=Inherit: Same as input  ParamDataTypeStr=Inherit: Same as input
  Math Function : Math  Operator=mod  OutDataType=sfix(16)  OutScaling=2^0  SaturateOnIntegerOverflow=on
  Math Function1 : Math  Operator=mod  OutDataType=sfix(16)  OutScaling=2^0  SaturateOnIntegerOverflow=on
  Sum1 : Sum  Inputs=|+-  OutDataType=sfix(16)  OutScaling=2^0  SaturateOnIntegerOverflow=on  InputSameDT=on  OutDataTypeStr=Inherit: Same as first input
  Sum2 : Sum  Inputs=|++  OutDataType=sfix(16)  OutScaling=2^0  SaturateOnIntegerOverflow=on  InputSameDT=on  OutDataTypeStr=Inherit: Same as first input
  Switch : Switch  Threshold=pi  SaturateOnIntegerOverflow=on  InputSameDT=on
  pi : Constant  Value=pi  OutDataType=sfix(16)  OutScaling=2^0
  pi/2 : Constant  Value=pi/2  OutDataType=sfix(16)  OutScaling=2^0
  Out : Outport  OutDataType=sfix(16)  OutScaling=2^0
  wires:
  2pi/1 -> Math Function1/2
  ChSign/1 -> Switch/1
  Sum2/1 -> Math Function1/1, Math Function/1
  In/1 -> Sum2/1
  Switch/1 -> Out/1
  Math Function1/1 -> Switch/2
  Sum1/1 -> Switch/3, ChSign/1
  pi/2/1 -> Sum2/2, Sum1/2
  Math Function/1 -> Sum1/1
  pi/1 -> Math Function/2

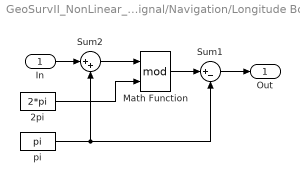
== system GeoSurvII_NonLinear_Signal/Navigation/Longitude Bound ==
  In : Inport  OutDataType=sfix(16)  OutScaling=2^0
  2pi : Constant  Value=2*pi  OutDataType=sfix(16)  OutScaling=2^0
  Math Function : Math  Operator=mod  OutDataType=sfix(16)  OutScaling=2^0  SaturateOnIntegerOverflow=on
  Sum1 : Sum  Inputs=|+-  OutDataType=sfix(16)  OutScaling=2^0  SaturateOnIntegerOverflow=on  InputSameDT=on  OutDataTypeStr=Inherit: Same as first input
  Sum2 : Sum  Inputs=|++  OutDataType=sfix(16)  OutScaling=2^0  SaturateOnIntegerOverflow=on  InputSameDT=on  OutDataTypeStr=Inherit: Same as first input
  pi : Constant  Value=pi  OutDataType=sfix(16)  OutScaling=2^0
  Out : Outport  OutDataType=sfix(16)  OutScaling=2^0
  wires:
  Math Function/1 -> Sum1/1
  2pi/1 -> Math Function/2
  In/1 -> Sum2/1
  Sum2/1 -> Math Function/1
  pi/1 -> Sum2/2, Sum1/2
  Sum1/1 -> Out/1

== matlab function GeoSurvII_NonLinear_EOM ==
  data: X input double; XDOT output double; U input double
function XDOT = Geo_model(X,U)

%GEO_MODEL Full 6 DOF model for GeoSurv II aircraft
%
%   [XDOT] = GEO_MODEL(X,U) returns the state derivatives, XDOT, given the
%   current state and inputs, X and U.  The constants are the nominal
%   constants.
%
%   State vector X and input vector U is defined as
%   
%       X = [u;v;w;p;q;r;phi;theta;psi] = [x1;x2;x3;x4;x5;x6;x7;x8;x9]
%       U = [d_A;d_E;d_R;d_th] = [u1;u2;u3;u4]
%
%
%Created by Christopher Lum
%lum@u.washington.edu
%Modified for GeoSurv II aircraft by Guillaume Blouin


%-----------------------CONSTANTS-------------------------------
%Unit conversions
lb_to_kg = 0.45359237;          %Unit conversion (pounds to kilograms)
in_to_m = 0.0254;               %Unit conversion (inches to meters)
ft_to_m = 0.3048;               %Unit conversion (feet to meters)
kt_to_ms = 0.514444;            %Unit conversion (knots to meters/second)
slug_to_kg = 14.593903;         %Unit conversion (slugs to kilograms)

%Mass moments of inertia
Ixx = 25.2589*slug_to_kg*ft_to_m^2;
Iyy = 32.8379*slug_to_kg*ft_to_m^2;
Izz = 47.0740*slug_to_kg*ft_to_m^2;
Ixz = 0*slug_to_kg*ft_to_m^2;

%Nominal vehicle constants (problem 1)
m = 186*lb_to_kg;               %Aircraft total mass (kg)
cbar = 27*in_to_m;              %Mean Aerodynamic Chord (m)
lt = 108.55*in_to_m;            %Distance by AC of tail and body (m)
S = 36*ft_to_m^2;               %Wing planform area (m^2)
St = 9.5*ft_to_m^2;             %Tail planform area (m^2)
i = -2*pi/180;                  %Tail incidence angle (rad)
AR = 7.11;                      %Aspect ratio
e = 0.836;                      %Oswalt's efficiency factor

Xcg = 0.25*cbar;                %x position of CoG in Fm (m)
Ycg = 0;                        %y position of CoG in Fm (m)
Zcg = 0.037*cbar;               %z position of CoG in Fm (m)

%Engine inputs
Xapt = 0;                       %x position of engine force in Fm (m)
Yapt = 0;                       %y position of engine force in Fm (m)
Zapt = 0.1405;                  %z position of engine force in Fm (m)

%Other constants
rho = 1.225;                    %Air density (kg/m^3)
g = 9.81;                       %Gravitational acceleration (m/s^2)
depsda = 0.33;                  %Change in downwash w.r.t. alpha (rad/rad)
alpha_L0 = -4*pi/180;           %Zero lift angle of attack (rad)

%Stability Derivatives (output from Justin Koning's Linear Model)
CXu = -0.096;
CXa = 0.19042;
CXadot = 0;
CXq = 0;
CXde = 0;
 
CZu = -1.0381;
CZa = -5.9345;
CZadot = -1.1763;
CZq = -5.6462;
CZde = -0.15543;
 
Cmu = 0;
Cma = -0.6094;
Cmadot = -4.496;
Cmq = -14.9865;
Cmde = -0.5958;
 
CYb = -0.5291;
CYbdot = 0;
CYp = 0.029801;
CYr = 0.4479;
CYda = 0;
CYdr = 0.13127;
 
Clb = -0.033192;
Clp = -0.49901;
Clr = 0.14677;
Clda = 0.14359;
Cldr = 0.0035059;
 
Cnb = 0.20878;
Cnbdot = 0;
Cnp = -0.071083;
Cnr = -0.20574;
Cnda = -0.0051955;
Cndr = -0.070618;

%Convert CZ to CL
CLu = -CZu;
CLa = -CZa;
CLadot = -CZadot;
CLq = -CZq;
CLde = -CZde;

%Other Stability Derivatives (from AERO database)
CDo = 0.0222;
CMo = -0.1003;
CLa_t = 3.544;


%--------------------------STATE VECTOR----------------------------------
%Extract state vector
x1 = X(1);                              %u
x2 = X(2);                              %v
x3 = X(3);                              %w
x4 = X(4);                              %p
x5 = X(5);                              %q
x6 = X(6);                              %r
x7 = X(7);                              %phi
x8 = X(8);                              %theta
x9 = X(9);                              %psi

u1 = U(1);                              %d_A (aileron)
u2 = U(2);                              %d_E (elevator)
u3 = U(3);                              %d_R (rudder)
u4 = U(4);                              %d_th (throttle)


%---------------INTERMEDIATE VARIABLES------------------------
%Calculate airspeed
Va = sqrt(x1^2 + x2^2 + x3^2);

%Calculate alpha and beta
alpha = atan(x3/x1);
beta = asin(x2/Va);

%Calculate dynamic pressure
Q = 0.5*rho*Va^2;

%Also define the vectors wbe_b and V_b 
wbe_b = [x4;x5;x6];
V_b = [x1;x2;x3];


%---------------AERODYNAMIC FORCE COEFFICIENTS----------------
%Calculate the CL_wb
if Va<(35.6*kt_to_ms)
end

if alpha<= 17*pi*180
    CL_wb=CLa*(alpha-alpha_L0);
elseif alpha>17*pi*180
    CL_wb=-5*10^-5*alpha^4+0.0034*alpha^3-0.092*alpha^2+1.1374*alpha-4.2971;
else
    CL_wb=2.75;
end

%Calculate CL_t
epsilon = depsda*(alpha - alpha_L0);
alpha_t = alpha - epsilon + i + CLq*x5*lt/Va;
CL_t = CLa_t*alpha_t + CLde*u2;

%Total lift force
CL = CL_wb + CL_t*(St/S);

%Total drag force (neglecting tail)
CD = CDo + CL^2/(pi*AR*e);

%Calculate sideforce
CY = CYb*beta + CYdr*u3 + CYr*x6;


%--------------DIMENSIONAL AERODYNAMIC FORCES---------------------
%Calculate the actual dimensional forces.  These are in F_s (stability axis)
FA_s = [-CD*Q*S;
         CY*Q*S;
        -CL*Q*S];
    
%Rotate these forces to F_b (body axis)
C_bs = [cos(alpha) 0 -sin(alpha);
        0 1 0;
        sin(alpha) 0 cos(alpha)];
    
FA_b = C_bs*FA_s;


%-------------AERODYNAMIC MOMENT COEFFICIENTS---------------
%Calculate the moments in Fb.  Define eta, dCMdx and dCMdu
eta11 = Clb*beta;
eta21 = CMo - (CLa_t*(St*lt)/(S*cbar))*(alpha - epsilon);
eta31 = Cnb*beta;

eta = [eta11;
       eta21;
       eta31];

dCMdx = (cbar/Va)*[Clp 0 Clr;
                    0 (Cmq*(St*lt^2)/(S*cbar^2)) 0;
                    Cnp 0 Cnr];
              
dCMdu = [Clda 0 Cldr;
          0 (-CLa_t*(St*lt)/(S*cbar)) 0;
          0 0 Cndr];

%Now calculate CM = [Cl;Cm;Cn] about Aerodynamic center in Fb
CMac_b = eta + dCMdx*wbe_b + dCMdu*[u1;u2;u3];

%Transfer now to CoG.
CX = -CD*cos(alpha) + CL*sin(alpha);
CZ = -CL*cos(alpha) - CD*sin(alpha);

A = (1/cbar)*[0 CZ -CY;
              -CZ 0 CX;
              CY -CX 0];

zeta = [(Xcg-0.12*cbar);
        -Ycg;
        Zcg];

CMcg_b = CMac_b + A*zeta;


%---------------DIMENSIONAL AERODYNAMIC MOMENTS---------------------
%Calculate the dimensional moments in Fb about cg
MAcg_b = CMcg_b*(Q*S*cbar);


%-----------------ENGINE FORCE & MOMENT----------------------------
%Now effect of engine.  First, calculate the thrust of engine
F = u4*m*g;

%Assuming that engine thrust is aligned with Fb, we have
FE_b = [F;0;0];
  
%Now engine moment due to offset of engine thrust from CoG.
mew = [Xcg - Xapt;
        Yapt - Ycg;
        Zcg - Zapt];


MEcg_b = cross(mew,FE_b);


%--------------------GRAVITY EFFECTS--------------------------------
%Calculate gravitational forces in the body frame.  This causes no moment
%about CoG.
g_b = [-g*sin(x8);
        g*cos(x8)*sin(x7);
        g*cos(x8)*cos(x7)];
  
Fg_b = m*g_b;


%-------------------STATE DERIVATIVES------------------------------
%Inertia matrix
Ib = m*[Ixx 0 Ixz;
        0 Iyy 0;
        Ixz 0 Izz];
    
%Inverse of inertia matrix 
invIb = inv(Ib);

%Form F_b (all the forces in Fb) and calculate udot, vdot, wdot
F_b = Fg_b + FE_b + FA_b;
x1to3dot = (1/m)*F_b - cross(wbe_b,V_b);

%Form Mcg_b (all moments about CoG in Fb) and calculate pdot, qdot, rdot.
Mcg_b = MAcg_b + MEcg_b;
x4to6dot = invIb*(Mcg_b - cross(wbe_b,Ib*wbe_b));

%Calculate phidot,thetadot, and psidot    
H_phi = [1 sin(x7)*tan(x8) cos(x7)*tan(x8);
         0 cos(x7) -sin(x7);
         0 sin(x7)/cos(x8) cos(x7)/cos(x8)];
    
x7to9dot = H_phi*wbe_b;

%Place in first order form
XDOT = [x1to3dot(1);                    %udot
        x1to3dot(2);                    %vdot
        x1to3dot(3);                    %wdot
        x4to6dot(1);                    %pdot
        x4to6dot(2);                    %qdot
        x4to6dot(3);                    %rdot
        x7to9dot(1);                    %phidot
        x7to9dot(2);                    %thetadot
        x7to9dot(3)];                   %psidot
